simulink model "slexAircraftExample"  (R2023a)
settings: Solver=ode45  StartTime=0.0  StopTime=60  RelTol=1e-4  AbsTol=1e-6
model workspace (MATLAB code in the model file):
  | slexAircraftData
values from neighbouring files (symbols this model uses):
  a = 2.5348    [slexAircraftData.m]
  b = 64.13    [slexAircraftData.m]
  Ka = 0.677    [slexAircraftData.m]
  Kf = -1.746    [slexAircraftData.m]
  Ki = -3.864    [slexAircraftData.m]
  Kq = 0.8156    [slexAircraftData.m]
  Md = -6.8847    [slexAircraftData.m]
  Mq = -0.6571    [slexAircraftData.m]
  Mw = -0.00592    [slexAircraftData.m]
  Swg = 3    [slexAircraftData.m]
  Ta = 0.05    [slexAircraftData.m]
  Tal = 0.3959    [slexAircraftData.m]
  Ts = 0.1    [slexAircraftData.m]
  Uo = 689.4    [slexAircraftData.m]
  Vto = 690.4    [slexAircraftData.m]
  W1 = 2.971    [slexAircraftData.m]
  W2 = 4.144    [slexAircraftData.m]
  Zd = -63.9979    [slexAircraftData.m]
  Zw = -0.6385    [slexAircraftData.m]
libraries: simulink x1
Description:
  | Aircraft Longitudinal Flight Control
  | 
  | This example shows how to model flight control for the longitudinal motion of an aircraft.
  | First order linear approximations of the aircraft and actuator behavior are connected
  | to an analog flight control design that uses the pilot's stick pitch command as the set point for the
  | aircraft's pitch attitude and uses aircraft pitch angle and pitch rate to determine commands.   A
  | simplified Dryden wind gust model is incorporated to perturb the system.
  | 
  | The Viewers and Generators Manager was used in this model to create the model scope for
  | viewing signals, Scope1.  Found on Simulation -> Prepare -> Viewers Manager, the Viewers and
  | Generators Manager allows you to instrument your model without having to add blocks to the
  | model.  If you close a model scope, such as for batch simulations, you can later reopen it
  | by double-clicking the "scope" icon on the signal of interest.
  | 
  | Parameters for the model are stored in a file named slexAircraftData.m.  This file is loaded
  | by the model into the model workspace.  You can view and edit data in the model workspace
  | directly by using the Model Explorer, which is launched using the Modeling -> Design
  | -> Model Explorer menu item.
settings Model: ModifiedByFormat=The MathWorks, Inc.  ExtModeTrigMode=oneshot  Creator=The MathWorks, Inc.  LastModifiedBy=The MathWorks, Inc.
settings SolverCC: AutoScaleAbsTol=off  AlgebraicLoopSolver=TrustRegion
settings DataIOCC: ExternalInput=[]  InitialState=[]  SaveFormat=Array  SaveState=on  ReturnWorkspaceOutputs=off
settings OptimizationCC: BlockReduction=off  BooleanDataType=off  ConditionallyExecuteInputs=off  OptimizeBlockIOStorage=off  BufferReuse=off  ReuseModelBlockBuffer=off  GlobalBufferReuse=off  ExpressionFolding=off  ExpressionDepthLimit=2147483647  LocalBlockOutputs=off  InitFltsAndDblsToZero=on  LifeSpan=inf  BufferReusableBoundary=off  OptimizeDataStoreBuffers=off  BusAssignmentInplaceUpdate=off
settings DebuggingCC: SaveWithParameterizedLinksMsg=none  SignalResolutionControl=TryResolveAllWithWarning  MultiTaskDSMMsg=warning  MultiTaskCondExecSysMsg=none  SigSpecEnsureSampleTimeMsg=none  IntegerOverflowMsg=none  FcnCallInpInsideContextMsg=warning  UnconnectedInputMsg=warning  UnconnectedOutputMsg=warning  UnconnectedLineMsg=warning  StateNameClashWarn=warning  SFUnexpectedBacktrackingDiag=warning  SFNoUnconditionalDefaultTransitionDiag=warning  SFExecutionAtInitializationDiag=none  IntegerSaturationMsg=none  ArithmeticOperatorsInVariantConditions=warning
settings HardwareCC: ProdBitPerPointer=32  ProdBitPerSizeT=32  ProdBitPerPtrDiffT=32  ProdLargestAtomicFloat=None  ProdIntDivRoundTo=Undefined  ProdEndianess=Unspecified  ProdWordSize=32  ProdHWDeviceType=32-bit Generic
settings ModelReferenceCC: EnableRefExpFcnMdlSchedulingChecks=on  PropagateSignalLabelsOutOfModel=off
settings SFSimCC: SimUseLocalCustomCode=off  CustomCodeUndefinedFunction=UseInterfaceOnly
settings RTWCC: RTWUseLocalCustomCode=off
settings CodeAppCC: StateflowObjectComments=on
settings GRTTargetCC: TargetFcnLib=ansi_tfl_tmw.mat  TargetLangStandard=C89/C90 (ANSI)  CombineOutputUpdateFcns=off  GRTInterface=on
settings ConfigComp: CovMetricSettings=dw  CovSaveCumulativeToWorkspaceVar=on  CovSaveSingleToWorkspaceVar=on  CovExternalEMLEnable=off

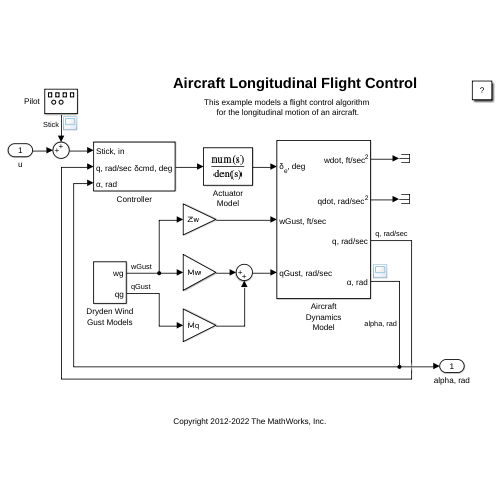
[thumbnail: Simulink's stored preview of the top-level diagram]
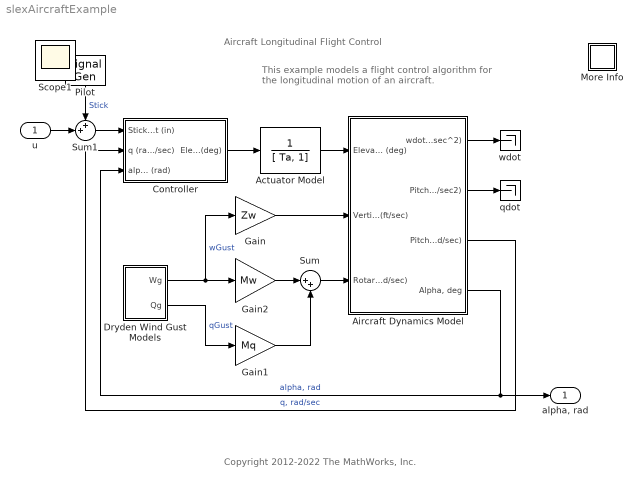
== system slexAircraftExample ==
  note: Aircraft Longitudinal Flight Control
  note: This example models a flight control algorithm
      | for the longitudinal motion of an aircraft.
  note: Copyright 2012-2022 The MathWorks, Inc.
  u : Inport
  Actuator Model : TransferFcn  Denominator=[ Ta, 1]
  Aircraft Dynamics Model : Subsystem
      mask Display:
      | port_label('input',1,'\delta_{e}, deg','texmode','on');
      | port_label('input',2,'wGust, ft/sec','texmode','on');
      | port_label('input',3,'qGust, rad/sec','texmode','on');
      | port_label('output',1,'wdot, ft/sec^2','texmode','on');
      | port_label('output',2,'qdot, rad/sec^{2}','texmode','on');
      | port_label('output',3,'q, rad/sec','texmode','on');
      | port_label('output',4,'\alpha, rad','texmode','on');
  Controller : Subsystem
      mask Display:
      | port_label('input',1,'Stick, in','texmode','on');
      | port_label('input',3,'\alpha, rad','texmode','on');
      | port_label('input',2,'q, rad/sec','texmode','on');
      | port_label('output',1,'\deltacmd, deg','texmode','on');
  Dryden Wind Gust Models : Subsystem
      mask Display:
      | port_label('output',1,'wg','texmode','on');
      | port_label('output',2,'qg','texmode','on');
  Gain : Gain  Gain=Zw  SaturateOnIntegerOverflow=on  OutDataTypeStr=Inherit: Same as input  ParamDataTypeStr=Inherit: Same as input
  Gain1 : Gain  Gain=Mq  SaturateOnIntegerOverflow=on  OutDataTypeStr=Inherit: Same as input  ParamDataTypeStr=Inherit: Same as input
  Gain2 : Gain  Gain=Mw  SaturateOnIntegerOverflow=on  OutDataTypeStr=Inherit: Same as input  ParamDataTypeStr=Inherit: Same as input
  More Info : Subsystem
      settings: OpenFcn=showExample('simulink_aerospace/AircraftLongitudinalFlightControlExample')
      mask Display: disp('?')
  Pilot : SignalGenerator  WaveForm=square  Amplitude=0.5  Frequency=0.500000  Units=rad/sec
  Sum : Sum  Inputs=|++  InputSameDT=on  SaturateOnIntegerOverflow=on  OutDataTypeStr=Inherit: Same as first input
  Sum1 : Sum  Inputs=++|  InputSameDT=on  SaturateOnIntegerOverflow=on  OutDataTypeStr=Inherit: Same as first input
  qdot : Terminator
  wdot : Terminator
  "alpha, rad" : Outport  InitialOutput=0  VectorParamsAs1DForOutWhenUnconnected=off
  Scope1 : Scope
  wires:
  Gain2/1 -> Sum/1
  Gain/1 -> Aircraft Dynamics Model/2(Vertical Gust wGust (ft/sec))
  Dryden Wind Gust Models/2(Qg) -> Gain1/1  "qGust"
  Dryden Wind Gust Models/1(Wg) -> Gain2/1, Gain/1  "wGust"
  Sum/1 -> Aircraft Dynamics Model/3(Rotary Gust qGust (rad/sec))
  Gain1/1 -> Sum/2
  Actuator Model/1 -> Aircraft Dynamics Model/1(Elevator Deflection d (deg))
  Controller/1(Elevator Command (deg)) -> Actuator Model/1
  Sum1/1 -> Controller/1(Stick Input (in))
  Pilot/1 -> Sum1/1  "Stick"
  u/1 -> Sum1/2
  Aircraft Dynamics Model/1(wdot (ft/sec^2)) -> wdot/1
  Aircraft Dynamics Model/2(Pitch Accel qdot (rad/sec2)) -> qdot/1
  Aircraft Dynamics Model/3(Pitch Rate q (rad/sec)) -> Controller/2(q (rad/sec))  "q, rad/sec"
  Aircraft Dynamics Model/4("Alpha, deg") -> Controller/3(alpha (rad)), "alpha, rad"/1  "alpha, rad"

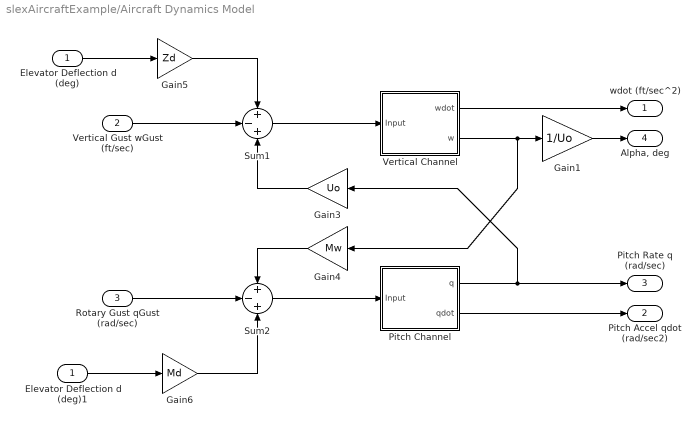
== system slexAircraftExample/Aircraft Dynamics Model ==
  Elevator Deflection d (deg) : Inport
  Vertical Gust wGust (ft/sec) : Inport  Port=2
  Rotary Gust qGust (rad/sec) : Inport  Port=3
  Elevator Deflection d (deg)1 : InportShadow
  Gain1 : Gain  Gain=1/Uo  SaturateOnIntegerOverflow=on  OutDataTypeStr=Inherit: Same as input  ParamDataTypeStr=Inherit: Same as input
  Gain3 : Gain  Gain=Uo  SaturateOnIntegerOverflow=on  OutDataTypeStr=Inherit: Same as input  ParamDataTypeStr=Inherit: Same as input
  Gain4 : Gain  Gain=Mw  SaturateOnIntegerOverflow=on  OutDataTypeStr=Inherit: Same as input  ParamDataTypeStr=Inherit: Same as input
  Gain5 : Gain  Gain=Zd  SaturateOnIntegerOverflow=on  OutDataTypeStr=Inherit: Same as input  ParamDataTypeStr=Inherit: Same as input
  Gain6 : Gain  Gain=Md  SaturateOnIntegerOverflow=on  OutDataTypeStr=Inherit: Same as input  ParamDataTypeStr=Inherit: Same as input
  Pitch Channel : Subsystem
  Sum1 : Sum  Inputs=+-+  InputSameDT=on  SaturateOnIntegerOverflow=on  OutDataTypeStr=Inherit: Same as first input
  Sum2 : Sum  Inputs=+-+  InputSameDT=on  SaturateOnIntegerOverflow=on  OutDataTypeStr=Inherit: Same as first input
  Vertical Channel : Subsystem
  wdot (ft/sec^2) : Outport  InitialOutput=0  VectorParamsAs1DForOutWhenUnconnected=off
  Pitch Accel qdot (rad/sec2) : Outport  Port=2  InitialOutput=0  VectorParamsAs1DForOutWhenUnconnected=off
  Pitch Rate q (rad/sec) : Outport  Port=3  InitialOutput=0  VectorParamsAs1DForOutWhenUnconnected=off
  "Alpha, deg" : Outport  Port=4  InitialOutput=0  VectorParamsAs1DForOutWhenUnconnected=off
  wires:
  Vertical Channel/2(w) -> Gain4/1, Gain1/1
  Pitch Channel/1(q) -> Pitch Rate q (rad/sec)/1, Gain3/1
  Gain6/1 -> Sum2/3
  Gain5/1 -> Sum1/1
  Gain3/1 -> Sum1/3
  Rotary Gust qGust (rad/sec)/1 -> Sum2/2
  Sum2/1 -> Pitch Channel/1(Input)
  Sum1/1 -> Vertical Channel/1(Input)
  Gain4/1 -> Sum2/1
  Vertical Gust wGust (ft/sec)/1 -> Sum1/2
  Elevator Deflection d (deg)/1 -> Gain5/1
  Elevator Deflection d (deg)1/1 -> Gain6/1
  Gain1/1 -> "Alpha, deg"/1
  Vertical Channel/1(wdot) -> wdot (ft/sec^2)/1
  Pitch Channel/2(qdot) -> Pitch Accel qdot (rad/sec2)/1

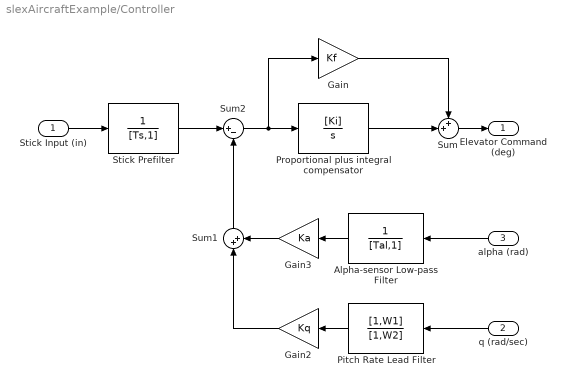
== system slexAircraftExample/Controller ==
  Stick Input (in) : Inport
  q (rad/sec) : Inport  Port=2
  alpha (rad) : Inport  Port=3
  Alpha-sensor Low-pass Filter : TransferFcn  Denominator=[Tal,1]
  Gain : Gain  Gain=Kf  SaturateOnIntegerOverflow=on  OutDataTypeStr=Inherit: Same as input  ParamDataTypeStr=Inherit: Same as input
  Gain2 : Gain  Gain=Kq  SaturateOnIntegerOverflow=on  OutDataTypeStr=Inherit: Same as input  ParamDataTypeStr=Inherit: Same as input
  Gain3 : Gain  Gain=Ka  SaturateOnIntegerOverflow=on  OutDataTypeStr=Inherit: Same as input  ParamDataTypeStr=Inherit: Same as input
  Pitch Rate Lead Filter : TransferFcn  Numerator=[1,W1]  Denominator=[1,W2]
  Proportional plus integral compensator : TransferFcn  Numerator=[Ki]  Denominator=[1,0]
  Stick Prefilter : TransferFcn  Denominator=[Ts,1]
  Sum : Sum  Inputs=++|  InputSameDT=on  SaturateOnIntegerOverflow=on  OutDataTypeStr=Inherit: Same as first input
  Sum1 : Sum  Inputs=|++  InputSameDT=on  SaturateOnIntegerOverflow=on  OutDataTypeStr=Inherit: Same as first input
  Sum2 : Sum  Inputs=|+-  InputSameDT=on  SaturateOnIntegerOverflow=on  OutDataTypeStr=Inherit: Same as first input
  Elevator Command (deg) : Outport  InitialOutput=0  VectorParamsAs1DForOutWhenUnconnected=off
  wires:
  Sum2/1 -> Proportional plus integral compensator/1, Gain/1
  Gain/1 -> Sum/1
  Proportional plus integral compensator/1 -> Sum/2
  Stick Prefilter/1 -> Sum2/1
  Sum/1 -> Elevator Command (deg)/1
  Gain2/1 -> Sum1/1
  Gain3/1 -> Sum1/2
  Sum1/1 -> Sum2/2
  Pitch Rate Lead Filter/1 -> Gain2/1
  q (rad/sec)/1 -> Pitch Rate Lead Filter/1
  Alpha-sensor Low-pass Filter/1 -> Gain3/1
  alpha (rad)/1 -> Alpha-sensor Low-pass Filter/1
  Stick Input (in)/1 -> Stick Prefilter/1

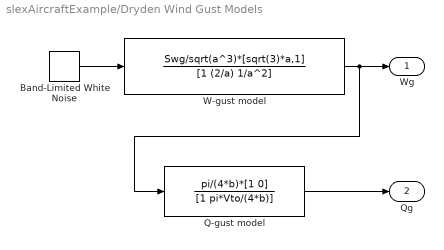
== system slexAircraftExample/Dryden Wind Gust Models ==
  Band-Limited White Noise : simulink/Sources/Band-Limited White Noise  Cov=1  Ts=0.1  seed=[23341]
  Q-gust model : TransferFcn  Numerator=pi/(4*b)*[1 0]  Denominator=[1 pi*Vto/(4*b)]
  W-gust model : TransferFcn  Numerator=Swg/sqrt(a^3)*[sqrt(3)*a,1]  Denominator=[1 (2/a) 1/a^2]
  Wg : Outport  InitialOutput=0  VectorParamsAs1DForOutWhenUnconnected=off
  Qg : Outport  Port=2  InitialOutput=0  VectorParamsAs1DForOutWhenUnconnected=off
  wires:
  Band-Limited White Noise/1 -> W-gust model/1
  Q-gust model/1 -> Qg/1
  W-gust model/1 -> Wg/1, Q-gust model/1

== system slexAircraftExample/More Info ==

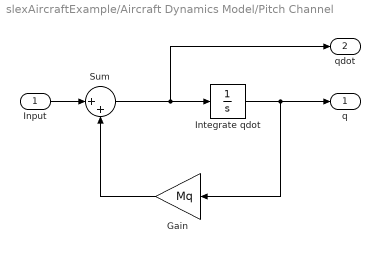
== system slexAircraftExample/Aircraft Dynamics Model/Pitch Channel ==
  Input : Inport
  Gain : Gain  Gain=Mq  SaturateOnIntegerOverflow=on  OutDataTypeStr=Inherit: Same as input  ParamDataTypeStr=Inherit: Same as input
  Integrate qdot : Integrator
  Sum : Sum  Inputs=|++  InputSameDT=on  SaturateOnIntegerOverflow=on  OutDataTypeStr=Inherit: Same as first input
  q : Outport  InitialOutput=0  VectorParamsAs1DForOutWhenUnconnected=off
  qdot : Outport  Port=2  InitialOutput=0  VectorParamsAs1DForOutWhenUnconnected=off
  wires:
  Sum/1 -> qdot/1, Integrate qdot/1
  Integrate qdot/1 -> Gain/1, q/1
  Gain/1 -> Sum/2
  Input/1 -> Sum/1

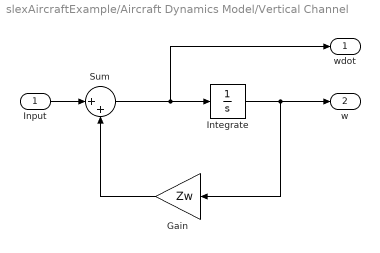
== system slexAircraftExample/Aircraft Dynamics Model/Vertical Channel ==
  Input : Inport
  Gain : Gain  Gain=Zw  SaturateOnIntegerOverflow=on  OutDataTypeStr=Inherit: Same as input  ParamDataTypeStr=Inherit: Same as input
  Integrate : Integrator
  Sum : Sum  Inputs=|++  InputSameDT=on  SaturateOnIntegerOverflow=on  OutDataTypeStr=Inherit: Same as first input
  wdot : Outport  InitialOutput=0  VectorParamsAs1DForOutWhenUnconnected=off
  w : Outport  Port=2  InitialOutput=0  VectorParamsAs1DForOutWhenUnconnected=off
  wires:
  Input/1 -> Sum/1
  Gain/1 -> Sum/2
  Integrate/1 -> w/1, Gain/1
  Sum/1 -> Integrate/1, wdot/1
